simulink model "svlvspr2_schema_SVLVS"  (R2018b)
settings: Solver=FixedStepAuto  StartTime=0.0  StopTime=Tsim  FixedStep=0.001  RelTol=1e-3
undefined symbols (not defined in the file): k, K, pidW
libraries: simulink x1
settings Model: Creator=Jan  LastModifiedBy=Jan

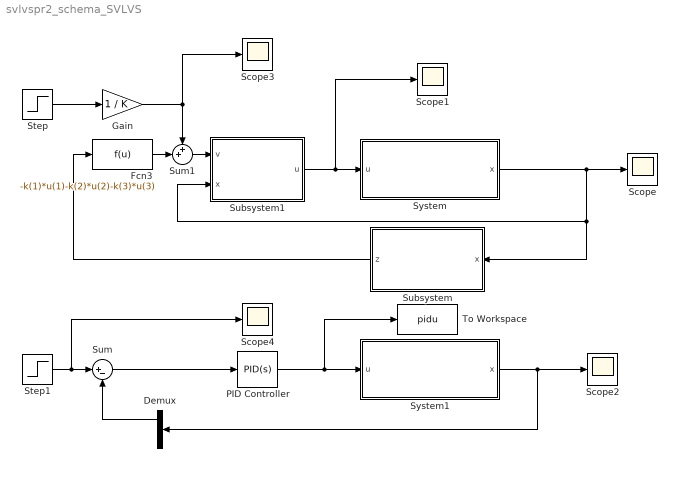
== system svlvspr2_schema_SVLVS ==
  Demux : Demux  Outputs=3
  Fcn3 : Fcn  Expr=-k(1)*u(1)-k(2)*u(2)-k(3)*u(3)
  Gain : Gain  Gain=1 / K
  PID Controller : simulink/Continuous/PID Controller  Controller=PID  Form=Parallel  TimeDomain=Continuous-time  SampleTime=-1  IntegratorMethod=Forward Euler  FilterMethod=Forward Euler  ControllerParametersSource=internal  P=1  I=0.25  D=1  UseFilter=on  N=100  TunerSelectOption=Transfer Function Based (PID Tuner App)  InitialConditionSource=internal  InitialConditionForIntegrator=0  InitialConditionForFilter=0  DifferentiatorICPrevScaledInput=0  ExternalReset=none  TrackingMode=off  Kt=1  LimitOutput=off  UpperSaturationLimit=inf  LowerSaturationLimit=-inf  LinearizeAsGain=on  AntiWindupMode=none  Kb=1  POutMin=[]  POutMax=[]  IOutMin=[]  IOutMax=[]  DOutMin=[]  DOutMax=[]  NOutMin=[]  NOutMax=[]  SumOutMin=[]  SumOutMax=[]  SaturationOutMin=[]  SaturationOutMax=[]  PParamMin=[]  PParamMax=[]  IParamMin=[]  IParamMax=[]  DParamMin=[]  DParamMax=[]  NParamMin=[]  NParamMax=[]  KbParamMin=[]  KbParamMax=[]  KtParamMin=[]  KtParamMax=[]  KbOutMin=[]  KbOutMax=[]  KtOutMin=[]  KtOutMax=[]  IntegratorOutMin=[]  IntegratorOutMax=[]  FilterOutMin=[]  FilterOutMax=[]  SumI1OutMin=[]  SumI1OutMax=[]  SumI2OutMin=[]  SumI2OutMax=[]  SumI3OutMin=[]  SumI3OutMax=[]  SumI4OutMin=[]  SumI4OutMax=[]  SumDOutMin=[]  SumDOutMax=[]  DifferentiatorOutMin=[]  DifferentiatorOutMax=[]  FilterDiffOutCoefMin=[]  FilterDiffOutCoefMax=[]  ReciprocalOutMin=[]  ReciprocalOutMax=[]  SumDenOutMin=[]  SumDenOutMax=[]  SumNumOutMin=[]  SumNumOutMax=[]  DivideOutMin=[]  DivideOutMax=[]  IntegratorContinuousStateAttributes=''  IntegratorStateMustResolveToSignalObject=off  IntegratorRTWStateStorageClass=Auto  FilterContinuousStateAttributes=''  FilterStateMustResolveToSignalObject=off  FilterRTWStateStorageClass=Auto  ParallelPVariant=InternalParameters  IdealPVariant=Disabled  IVariant=InternalParameters  DVariant=InternalParameters  IntegratorVariant=Continuous  SatVariant=Disabled  AWVariant=Passthrough  PCopyVariant=Disabled  TRVariant=Disabled  FdbkBlocksVariant=Forward  IdealPFdbkVariant=Disabled  SatFdbkVariant=Disabled  DerivativeFilterVariant=ContFilter  NVariant=InternalParameters  NCopyVariant=Disabled  FilterICVariant=InternalICsFilter  IntegratorICVariant=InternalICs  ExternalResetVariant=Disabled  TRSumVariant=Passthrough  SumFdbkVariant=Disabled  SumVariant=Sum_PID
  Scope{,1..4} (5 alike) : Scope
  Step : Step  Time=0  After=10  SampleTime=0
  Step1 : Step  Time=0  After=pidW  SampleTime=0
  Subsystem : Subsystem
  Subsystem1 : Subsystem
  Sum : Sum  Inputs=|+-
  Sum1 : Sum  Inputs=++|
  System : Subsystem
  System1 : Subsystem
  To Workspace : ToWorkspace  VariableName=pidu  SaveFormat=Timeseries  SampleTime=-1
  wires:
  Subsystem1/1(u) -> Scope1/1, System/1(u)
  System/1(x) -> Scope/1, Subsystem/1(x), Subsystem1/2(x)
  Step/1 -> Gain/1
  Sum1/1 -> Subsystem1/1(v)
  Fcn3/1 -> Sum1/2
  Subsystem/1(z) -> Fcn3/1
  Gain/1 -> Scope3/1, Sum1/1
  System1/1(x) -> Demux/1, Scope2/1
  Sum/1 -> PID Controller/1
  PID Controller/1 -> To Workspace/1, System1/1(u)
  Step1/1 -> Scope4/1, Sum/1
  Demux/1 -> Sum/2

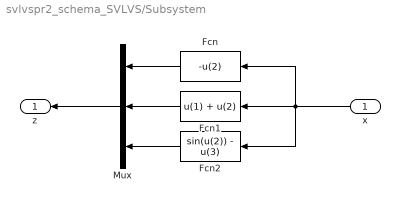
== system svlvspr2_schema_SVLVS/Subsystem ==
  x : Inport
  Fcn : Fcn  Expr=-u(2)
  Fcn1 : Fcn  Expr=u(1) + u(2)
  Fcn2 : Fcn  Expr=sin(u(2)) - u(3)
  Mux : Mux  Inputs=3
  z : Outport
  wires:
  Fcn/1 -> Mux/1
  Fcn2/1 -> Mux/3
  Fcn1/1 -> Mux/2
  Mux/1 -> z/1
  x/1 -> Fcn2/1, Fcn/1, Fcn1/1

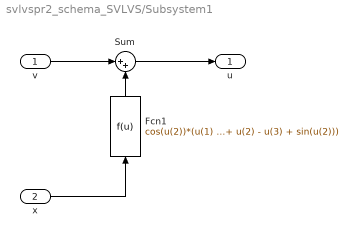
== system svlvspr2_schema_SVLVS/Subsystem1 ==
  v : Inport
  x : Inport  Port=2
  Fcn1 : Fcn  Expr=cos(u(2))*(u(1) + u(2) - u(3) + sin(u(2)))
  Sum : Sum  Inputs=|++
  u : Outport
  wires:
  Fcn1/1 -> Sum/2
  v/1 -> Sum/1
  Sum/1 -> u/1
  x/1 -> Fcn1/1

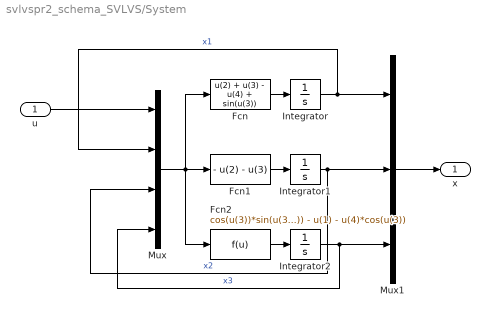
== system svlvspr2_schema_SVLVS/System ==
  u : Inport
  Fcn : Fcn  Expr=u(2) + u(3) - u(4) + sin(u(3))
  Fcn1 : Fcn  Expr=- u(2) - u(3)
  Fcn2 : Fcn  Expr=cos(u(3))*sin(u(3)) - u(1) - u(4)*cos(u(3))
  Integrator : Integrator
  Integrator1 : Integrator
  Integrator2 : Integrator
  Mux : Mux
  Mux1 : Mux  Inputs=3
  x : Outport
  wires:
  u/1 -> Mux/1
  Integrator1/1 -> Mux/3, Mux1/2  "x2"
  Mux/1 -> Fcn/1, Fcn1/1, Fcn2/1
  Integrator/1 -> Mux/2, Mux1/1  "x1"
  Fcn/1 -> Integrator/1
  Fcn1/1 -> Integrator1/1
  Fcn2/1 -> Integrator2/1
  Integrator2/1 -> Mux/4, Mux1/3  "x3"
  Mux1/1 -> x/1

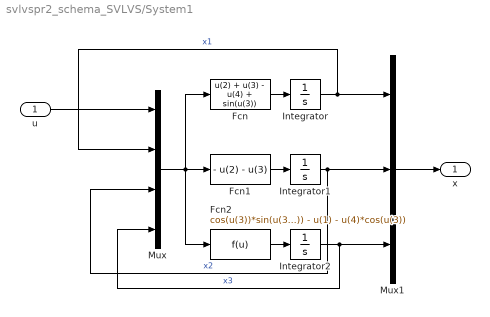
== system svlvspr2_schema_SVLVS/System1 ==
  u : Inport
  Fcn : Fcn  Expr=u(2) + u(3) - u(4) + sin(u(3))
  Fcn1 : Fcn  Expr=- u(2) - u(3)
  Fcn2 : Fcn  Expr=cos(u(3))*sin(u(3)) - u(1) - u(4)*cos(u(3))
  Integrator : Integrator
  Integrator1 : Integrator
  Integrator2 : Integrator
  Mux : Mux
  Mux1 : Mux  Inputs=3
  x : Outport
  wires:
  Mux1/1 -> x/1
  Integrator2/1 -> Mux1/3, Mux/4  "x3"
  Fcn2/1 -> Integrator2/1
  Fcn1/1 -> Integrator1/1
  Fcn/1 -> Integrator/1
  Integrator/1 -> Mux1/1, Mux/2  "x1"
  Mux/1 -> Fcn2/1, Fcn1/1, Fcn/1
  Integrator1/1 -> Mux1/2, Mux/3  "x2"
  u/1 -> Mux/1
